simulink model "PID_model_comparison"  (R2016b)
settings: Solver=FixedStepAuto  StartTime=0.0  StopTime=10  FixedStep=Ts  RelTol=1e-3  EnableMultiTasking=on
PreLoadFcn:
  | load('ModelParameters.mat')
StartFcn:
  | Ts=0.03
libraries: simulink x1
settings Model: ExtModeTrigDuration=5  Creator=AlexandrY  LastModifiedBy=AlexandrY
settings SolverCC: AutoInsertRateTranBlk=on
settings OptimizationCC: DefaultParameterBehavior=Inlined  UseDivisionForNetSlopeComputation=on  UseFloatMulNetSlope=on  InlineInvariantSignals=on  PassReuseOutputArgsAs=Individual arguments  ZeroExternalMemoryAtStartup=off  ZeroInternalMemoryAtStartup=off  NoFixptDivByZeroProtection=on  EfficientFloat2IntCast=on  LifeSpan=1  MaxStackSize=64
settings DebuggingCC: ParameterTunabilityLossMsg=error  BusObjectLabelMismatch=error
settings HardwareCC: ProdBitPerPointer=32  ProdBitPerSizeT=32  ProdBitPerPtrDiffT=32  ProdLargestAtomicInteger=Long  ProdLargestAtomicFloat=Double  ProdWordSize=32  ProdHWDeviceType=ARM Compatible->ARM Cortex
settings RTWCC: SystemTargetFile=ert.tlc  HardwareBoard=NXP FRDM-K64F  TLCOptions="-aInlineSetEventsForThisBaseRateFcn=TLC_FALSE -aSuppressMultiTaskScheduler=TLC_FALSE  -aRateBasedStepFcn=0"  PackageGeneratedCodeAndArtifacts=on  PackageName=GeneratedCode  TemplateMakefile=ert_default_tmf  Description=Embedded Coder  GenerateReport=on  Toolchain=GNU Tools for ARM Embedded Processors  BuildConfiguration=Debug  IncludeHyperlinkInReport=on  LaunchReport=on  GenerateTraceInfo=on  GenerateTraceReport=on  GenerateTraceReportSl=on  GenerateTraceReportSf=on  GenerateTraceReportEml=on  GenerateCodeMetricsReport=on
settings CodeAppCC: ForceParamTrailComments=on  CommentStyle=Single-line  IgnoreCustomStorageClasses=off  OperatorAnnotations=on  SimulinkDataObjDesc=on  SFDataObjDesc=on  MATLABFcnDesc=on  CustomSymbolStrGlobalVar=rt$N$M  CustomSymbolStrType=$N$M  CustomSymbolStrFcn=$N$M$F  CustomSymbolStrMacro=$N$M  InsertBlockDesc=on  MATLABSourceComments=on  EnableCustomComments=on  ReqsInCode=on
settings ERTTargetCC: CodeReplacementLibrary=ARM Cortex-M (Optimized)  IncludeMdlTerminateFcn=off  CombineSignalStateStructs=on  MultiInstanceERTCode=on  CodeInterfacePackaging=Reusable function  SupportComplex=off  SupportNonInlinedSFcns=on  ParenthesesLevel=Maximum  InlinedParameterPlacement=NonHierarchical  RootIOFormat=Structure reference  ERTFilePackagingFormat=CompactWithDataFile  ConvertIfToSwitch=off  IndentStyle=Allman

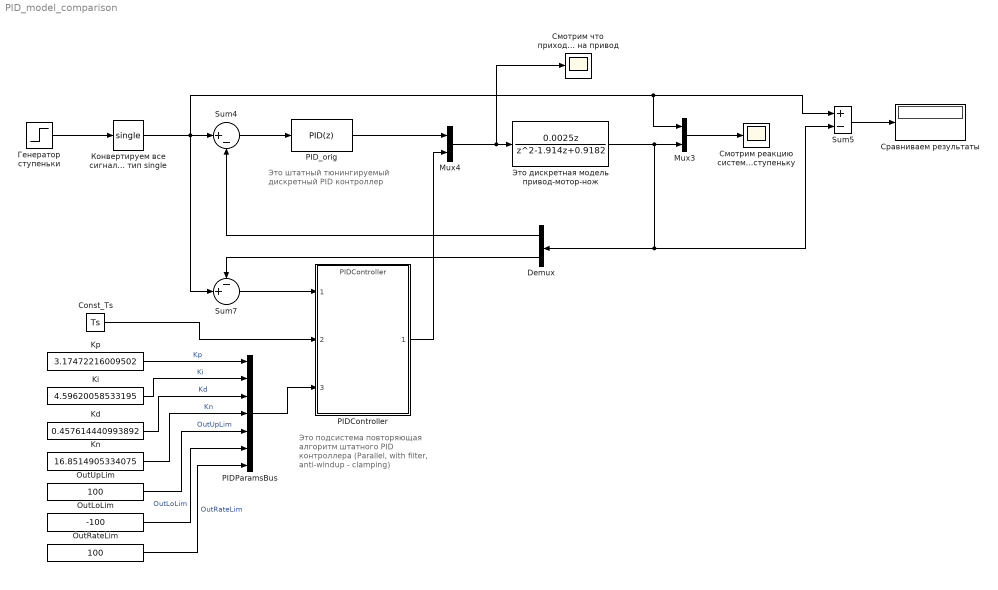
== system PID_model_comparison ==
  note: Это подсистема повторяющая
      | алгоритм штатного
      | PID контроллера (Parallel, with filter, anti-windup - clamping)
  note: Это штатный тюнингируемый
      | дискретный PID контроллер
  Const_Ts : Constant  DisableCoverage=on  Value=Ts  OutDataTypeStr=single  SampleTime=-1  PreserveConstantTs=on
  Demux : Demux  Outputs=2
  Kd : Constant  DisableCoverage=on  Value=0.457614440993892  OutDataTypeStr=Inherit: Inherit via back propagation  SampleTime=Ts  PreserveConstantTs=on
  Ki : Constant  DisableCoverage=on  Value=4.59620058533195  OutDataTypeStr=Inherit: Inherit via back propagation  SampleTime=Ts  PreserveConstantTs=on
  Kn : Constant  DisableCoverage=on  Value=16.8514905334075  OutDataTypeStr=Inherit: Inherit via back propagation  SampleTime=Ts  PreserveConstantTs=on
  Kp : Constant  DisableCoverage=on  Value=3.17472216009502  OutDataTypeStr=Inherit: Inherit via back propagation  SampleTime=Ts  PreserveConstantTs=on
  Mux3 : Mux  Inputs=2
  Mux4 : Mux  Inputs=2
  OutLoLim : Constant  DisableCoverage=on  Value=-100  OutDataTypeStr=Inherit: Inherit via back propagation  SampleTime=Ts  PreserveConstantTs=on
  OutRateLim : Constant  DisableCoverage=on  Value=100  OutDataTypeStr=Inherit: Inherit via back propagation  SampleTime=Ts  PreserveConstantTs=on
  OutUpLim : Constant  DisableCoverage=on  Value=100  OutDataTypeStr=Inherit: Inherit via back propagation  SampleTime=Ts  PreserveConstantTs=on
  PIDController : ModelReference  ModelNameDialog=PIDController  SimulationMode=Normal  ModelReferenceVersion=1.77
  PIDParamsBus : BusCreator  Inputs='Kp','Ki','Kd','Kn','OutUpLim','OutLoLim','OutRateLim'  OutDataTypeStr=Bus: PIDParams
  PID_orig : simulink/Continuous/PID Controller  Controller=PID  TimeDomain=Discrete-time  SampleTime=-1  IntegratorMethod=Forward Euler  FilterMethod=Forward Euler  Form=Parallel  UseFilter=on  ControllerParametersSource=internal  P=3.17472216009502  I=4.59620058533195  D=0.457614440993892  N=16.8514905334075  InitialConditionSource=internal  InitialConditionForIntegrator=0  InitialConditionForFilter=0  ExternalReset=none  LimitOutput=on  UpperSaturationLimit=100  LowerSaturationLimit=-100  LinearizeAsGain=off  AntiWindupMode=clamping  Kb=4  TrackingMode=off  Kt=1  PParamMin=[]  PParamMax=[]  PParamDataTypeStr=single  IParamMin=[]  IParamMax=[]  IParamDataTypeStr=single  DParamMin=[]  DParamMax=[]  DParamDataTypeStr=single  NParamMin=[]  NParamMax=[]  NParamDataTypeStr=single  KbParamMin=[]  KbParamMax=[]  KtParamMin=[]  KtParamMax=[]  POutMin=[]  POutMax=[]  POutDataTypeStr=single  PGainOutDataTypeStr=single  PProdOutDataTypeStr=single  IOutMin=[]  IOutMax=[]  IOutDataTypeStr=single  IGainOutDataTypeStr=single  IProdOutDataTypeStr=single  DOutMin=[]  DOutMax=[]  DOutDataTypeStr=single  DGainOutDataTypeStr=single  DProdOutDataTypeStr=single  NOutMin=[]  NOutMax=[]  NOutDataTypeStr=single  NGainOutDataTypeStr=single  NProdOutDataTypeStr=single  KbOutMin=[]  KbOutMax=[]  KtOutMin=[]  KtOutMax=[]  IntegratorOutMin=[]  IntegratorOutMax=[]  IntegratorOutDataTypeStr=single  FilterOutMin=[]  FilterOutMax=[]  FilterOutDataTypeStr=single  SumOutMin=[]  SumOutMax=[]  SumOutDataTypeStr=single  SumI1OutMin=[]  SumI1OutMax=[]  SumI2OutMin=[]  SumI2OutMax=[]  SumI3OutMin=[]  SumI3OutMax=[]  SumDOutMin=[]  SumDOutMax=[]  SumDOutDataTypeStr=single  SumAccumDataTypeStr=single  SumDAccumDataTypeStr=single  SaturationOutMin=[]  SaturationOutMax=[]  IntegratorContinuousStateAttributes=''  IntegratorStateMustResolveToSignalObject=off  IntegratorRTWStateStorageClass=Auto  FilterContinuousStateAttributes=''  FilterStateMustResolveToSignalObject=off  FilterRTWStateStorageClass=Auto  DifferentiatorICPrevScaledInput=0  DifferentiatorOutMin=[]  DifferentiatorOutMax=[]
  Sum4 : Sum  Inputs=|+-
  Sum5 : Sum  Inputs=+-
  Sum7 : Sum  Inputs=-+|
  Генератор ступеньки : Step  After=15  SampleTime=Ts
  "Конвертируем все сигналы модели в тип single " : DataTypeConversion  OutDataTypeStr=single
  Смотрим реакцию системы на ступеньку : Scope
  Смотрим что приходит на привод : Scope
  "Сравниваем результаты " : Display
  Это дискретная модель привод-мотор-нож : DiscreteTransferFcn  Numerator=[0.0025 0]  Denominator=[1 -1.914 0.9182]
  wires:
  Генератор ступеньки/1 -> "Конвертируем все сигналы модели в тип single "/1
  Sum4/1 -> PID_orig/1
  PID_orig/1 -> Mux4/1
  "Конвертируем все сигналы модели в тип single "/1 -> Sum5/1, Mux3/1, Sum7/2, Sum4/1
  Это дискретная модель привод-мотор-нож/1 -> Mux3/2, Demux/1, Sum5/2
  Mux3/1 -> Смотрим реакцию системы на ступеньку/1
  Sum5/1 -> "Сравниваем результаты "/1
  Mux4/1 -> Это дискретная модель привод-мотор-нож/1, Смотрим что приходит на привод/1
  Demux/1 -> Sum4/2
  Sum7/1 -> PIDController/1
  PIDController/1 -> Mux4/2
  Demux/2 -> Sum7/1
  Kp/1 -> PIDParamsBus/1  "Kp"
  Ki/1 -> PIDParamsBus/2  "Ki"
  Kd/1 -> PIDParamsBus/3  "Kd"
  Kn/1 -> PIDParamsBus/4  "Kn"
  OutUpLim/1 -> PIDParamsBus/5  "OutUpLim"
  OutLoLim/1 -> PIDParamsBus/6  "OutLoLim"
  OutRateLim/1 -> PIDParamsBus/7  "OutRateLim"
  PIDParamsBus/1 -> PIDController/3
  Const_Ts/1 -> PIDController/2
